simulink model "CarControl"  (R2018a)
settings: Solver=VariableStepAuto  StartTime=0.0  StopTime=5  RelTol=1e-8
libraries: fuzblock x1, simulink x1
settings Model: Creator=Nikos  LastModifiedBy=Nikos
settings SolverCC: AlgebraicLoopSolver=LineSearch

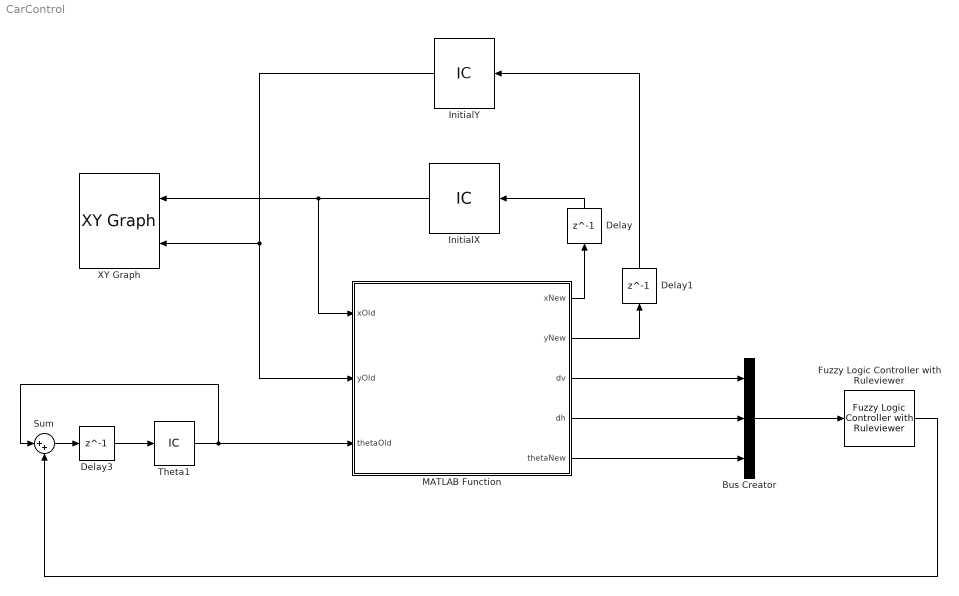
== system CarControl ==
  Bus Creator : BusCreator  Inputs=3
  Delay : Delay  DelayLength=1  InitialCondition=0
  Delay1 : Delay  DelayLength=1  InitialCondition=0
  Delay3 : Delay  DelayLength=1  InitialCondition=0
  Fuzzy Logic Controller with Ruleviewer : fuzblock/Fuzzy Logic  Controller  with Ruleviewer  fismatrix=FLCCarSim  Ts=0.01
  InitialX : InitialCondition  Value=4.1
  InitialY : InitialCondition  Value=0.3
  MATLAB Function : MATLAB Function  TreatAsAtomicUnit=on
  Sum : Sum  Inputs=|++
  Theta1 : InitialCondition  Value=0
  XY Graph : simulink/Sinks/XY Graph  xmin=0  xmax=10  ymin=0  ymax=4  st=-1
  wires:
  MATLAB Function/1(xNew) -> Delay/1
  MATLAB Function/3(dv) -> Bus Creator/1
  MATLAB Function/4(dh) -> Bus Creator/2
  MATLAB Function/5(thetaNew) -> Bus Creator/3
  InitialX/1 -> XY Graph/1, MATLAB Function/1(xOld)
  MATLAB Function/2(yNew) -> Delay1/1
  InitialY/1 -> XY Graph/2, MATLAB Function/2(yOld)
  Bus Creator/1 -> Fuzzy Logic Controller with Ruleviewer/1
  Delay1/1 -> InitialY/1
  Delay/1 -> InitialX/1
  Fuzzy Logic Controller with Ruleviewer/1 -> Sum/2
  Theta1/1 -> Sum/1, MATLAB Function/3(thetaOld)
  Sum/1 -> Delay3/1
  Delay3/1 -> Theta1/1

== matlab function CarControl/MATLAB Function ==
  data: xOld input; xNew output; yOld input; thetaOld input; yNew output; dv output; dh output; thetaNew output
function [xNew,yNew,dv,dh,thetaNew]= fcn(xOld,yOld,thetaOld)
    theta = thetaOld;
    thetaNew = theta;
    thetaRadians = theta/360*2*pi;
    
    if( theta < -180 )
        theta = -180;
    end
    
    if( theta > 180 )
        theta = 180;
    end
    
    
    % calculate new coordinates
    u = 0.05;
    dx = u * cos(thetaRadians);
    dy = u * sin(thetaRadians);
    
    dv = 0;
    dh = 0;
    
    xNew = xOld + dx;
    yNew = yOld + dy;
    
    % calculate dv and dh
    if( xNew < 5 )
        dv = yNew;
    elseif( xNew < 6 )
        dv = yNew - 1;
    elseif( xNew < 7 )
        dv = yNew - 2;
    else
        dv = yNew - 3;
    end
    
    if( yNew < 1 )
        dh = 5 - xNew;
    elseif( yNew < 2 )
        dh = 6 - xNew;
    elseif( yNew <  3 )
        dh = 7 - xNew;
    else
        dh = 1;
    end
    
    
    if( dv > 1 )
        dv = 1;
    end
    
    if( dv < 0 )
        dv = 0;
    end
    
    if( dh > 1 )
        dh = 1;
    end
    
    if( dh < 0 )
        dh = 0;
    end
    
end
